simulink model "PID_Tune"  (R2021b)
settings: Solver=FixedStepAuto  StartTime=0.0  StopTime=20  FixedStep=0.1  RelTol=1e-3
values from neighbouring files (symbols this model uses):
  inner_h = 0.1    [dataset.mat]    (also in initiateVars.m; system_workspace.mat; system_workspace_ayk.mat)
  omega_max_lim = 2500    [dataset.mat]    (also in initiateVars.m; system_workspace.mat; system_workspace_ayk.mat)
  omega_min_lim = 0    [dataset.mat]    (also in initiateVars.m; system_workspace.mat; system_workspace_ayk.mat)
  T_max_lim = 0.495    [dataset.mat]    (also in initiateVars.m = Tp - (Tp - Tm) * sat_lim; system_workspace.mat; system_workspace_ayk.mat)
  T_min_lim = 0.055    [dataset.mat]    (also in initiateVars.m = Tm + (Tp - Tm) * sat_lim; system_workspace.mat; system_workspace_ayk.mat)
  tau_max_lim = 1e-05    [dataset.mat]    (also in initiateVars.m; system_workspace.mat; system_workspace_ayk.mat)
  tau_min_lim = -1e-05    [dataset.mat]    (also in initiateVars.m; system_workspace.mat; system_workspace_ayk.mat)
libraries: slpidlib x2
settings Model: Creator=fethi  LastModifiedBy=fethi
settings SolverCC: AlgebraicLoopSolver=TrustRegion
settings DebuggingCC: SFMachineParentedDataDiag=warning

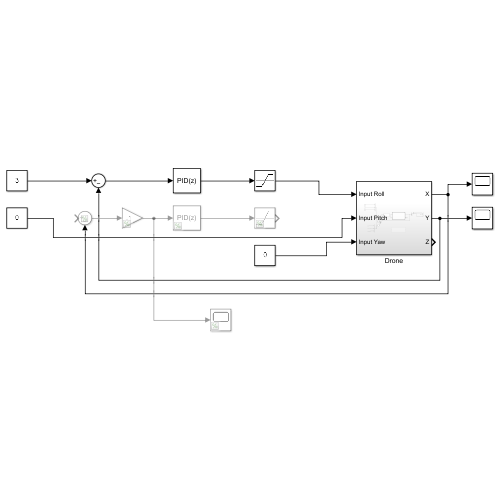
[thumbnail: Simulink's stored preview of the top-level diagram]
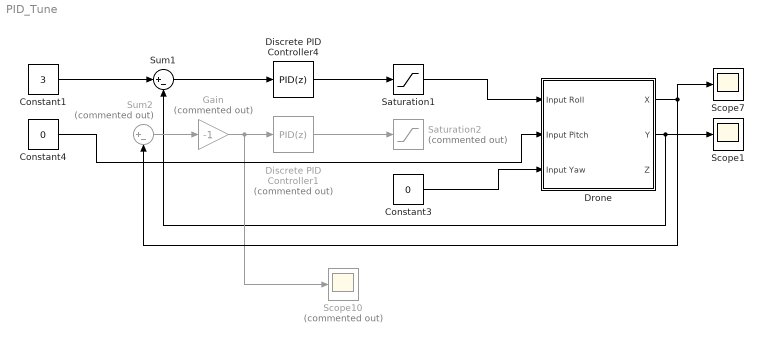
== system PID_Tune ==
  Constant1 : Constant  Value=3
  Constant3 : Constant  Value=0
  Constant4 : Constant  Value=0
  Discrete PID Controller1 : slpidlib/PID Controller  Commented=on  Controller=PID  Form=Parallel  TimeDomain=Discrete-time  UseExternalTs=off  SampleTime=-1  IntegratorMethod=Forward Euler  FilterMethod=Forward Euler  ControllerParametersSource=internal  P=-0.034  I=-8.37942170328314e-06  D=-0.0838262219971284  UseFilter=on  N=16.4387565401463  TunerSelectOption=Transfer Function Based (PID Tuner App)  InitialConditionSource=internal  InitialConditionForIntegrator=0  InitialConditionForFilter=0  DifferentiatorICPrevScaledInput=0  ExternalReset=none  TrackingMode=off  Kt=1  LimitOutput=off  SatLimitsSource=internal  UpperSaturationLimit=inf  LowerSaturationLimit=-inf  LinearizeAsGain=off  AntiWindupMode=none  Kb=1  POutMin=[]  POutMax=[]  IOutMin=[]  IOutMax=[]  DOutMin=[]  DOutMax=[]  NOutMin=[]  NOutMax=[]  SumOutMin=[]  SumOutMax=[]  SaturationOutMin=[]  SaturationOutMax=[]  PParamMin=[]  PParamMax=[]  IParamMin=[]  IParamMax=[]  DParamMin=[]  DParamMax=[]  NParamMin=[]  NParamMax=[]  KbParamMin=[]  KbParamMax=[]  KtParamMin=[]  KtParamMax=[]  KbOutMin=[]  KbOutMax=[]  KtOutMin=[]  KtOutMax=[]  IntegratorOutMin=[]  IntegratorOutMax=[]  FilterOutMin=[]  FilterOutMax=[]  SumI1OutMin=[]  SumI1OutMax=[]  SumI2OutMin=[]  SumI2OutMax=[]  SumI3OutMin=[]  SumI3OutMax=[]  SumI4OutMin=[]  SumI4OutMax=[]  SumDOutMin=[]  SumDOutMax=[]  DifferentiatorOutMin=[]  DifferentiatorOutMax=[]  FilterDiffOutCoefMin=[]  FilterDiffOutCoefMax=[]  ReciprocalOutMin=[]  ReciprocalOutMax=[]  SumDenOutMin=[]  SumDenOutMax=[]  SumNumOutMin=[]  SumNumOutMax=[]  DivideOutMin=[]  DivideOutMax=[]  UdiffTsProdOutMin=[]  UdiffTsProdOutMax=[]  NTsProdOutMin=[]  NTsProdOutMax=[]  UintegralTsProdOutMin=[]  UintegralTsProdOutMax=[]  UngainTsProdOutMin=[]  UngainTsProdOutMax=[]  IntegratorContinuousStateAttributes=''  IntegratorStateMustResolveToSignalObject=off  IntegratorRTWStateStorageClass=Auto  FilterContinuousStateAttributes=''  FilterStateMustResolveToSignalObject=off  FilterRTWStateStorageClass=Auto  ParallelPVariant=InternalParameters  IdealPVariant=Disabled  IVariant=InternalParameters  DVariant=InternalParameters  IntegratorVariant=Discrete  SatVariant=Disabled  AWVariant=Passthrough  PCopyVariant=Disabled  TRVariant=Disabled  FdbkBlocksVariant=Forward  IdealPFdbkVariant=Disabled  SatFdbkVariant=Disabled  DerivativeFilterVariant=ForwardEulerFilter  NVariant=InternalParameters  NCopyVariant=Disabled  FilterICVariant=InternalICsFilter  IntegratorICVariant=InternalICs  ExternalResetVariant=Disabled  TRSumVariant=Passthrough  SumFdbkVariant=Disabled  SumVariant=Sum_PID  TsampFilterVariant=InternalTs  TsampNgainVariant=Passthrough  TsampIntegralVariant=Passthrough  ExternalSaturationOutDataTypeStr=Inherit: Same as second input
  Discrete PID Controller4 : slpidlib/PID Controller  Controller=PID  Form=Parallel  TimeDomain=Discrete-time  UseExternalTs=off  SampleTime=-1  IntegratorMethod=Forward Euler  FilterMethod=Forward Euler  ControllerParametersSource=internal  P=-0.034  I=-8.37942170328314e-06  D=-0.0838262219971284  UseFilter=on  N=16.4387565401463  TunerSelectOption=Transfer Function Based (PID Tuner App)  InitialConditionSource=internal  InitialConditionForIntegrator=0  InitialConditionForFilter=0  DifferentiatorICPrevScaledInput=0  ExternalReset=none  TrackingMode=off  Kt=1  LimitOutput=off  SatLimitsSource=internal  UpperSaturationLimit=inf  LowerSaturationLimit=-inf  LinearizeAsGain=off  AntiWindupMode=none  Kb=1  POutMin=[]  POutMax=[]  IOutMin=[]  IOutMax=[]  DOutMin=[]  DOutMax=[]  NOutMin=[]  NOutMax=[]  SumOutMin=[]  SumOutMax=[]  SaturationOutMin=[]  SaturationOutMax=[]  PParamMin=[]  PParamMax=[]  IParamMin=[]  IParamMax=[]  DParamMin=[]  DParamMax=[]  NParamMin=[]  NParamMax=[]  KbParamMin=[]  KbParamMax=[]  KtParamMin=[]  KtParamMax=[]  KbOutMin=[]  KbOutMax=[]  KtOutMin=[]  KtOutMax=[]  IntegratorOutMin=[]  IntegratorOutMax=[]  FilterOutMin=[]  FilterOutMax=[]  SumI1OutMin=[]  SumI1OutMax=[]  SumI2OutMin=[]  SumI2OutMax=[]  SumI3OutMin=[]  SumI3OutMax=[]  SumI4OutMin=[]  SumI4OutMax=[]  SumDOutMin=[]  SumDOutMax=[]  DifferentiatorOutMin=[]  DifferentiatorOutMax=[]  FilterDiffOutCoefMin=[]  FilterDiffOutCoefMax=[]  ReciprocalOutMin=[]  ReciprocalOutMax=[]  SumDenOutMin=[]  SumDenOutMax=[]  SumNumOutMin=[]  SumNumOutMax=[]  DivideOutMin=[]  DivideOutMax=[]  UdiffTsProdOutMin=[]  UdiffTsProdOutMax=[]  NTsProdOutMin=[]  NTsProdOutMax=[]  UintegralTsProdOutMin=[]  UintegralTsProdOutMax=[]  UngainTsProdOutMin=[]  UngainTsProdOutMax=[]  IntegratorContinuousStateAttributes=''  IntegratorStateMustResolveToSignalObject=off  IntegratorRTWStateStorageClass=Auto  FilterContinuousStateAttributes=''  FilterStateMustResolveToSignalObject=off  FilterRTWStateStorageClass=Auto  ParallelPVariant=InternalParameters  IdealPVariant=Disabled  IVariant=InternalParameters  DVariant=InternalParameters  IntegratorVariant=Discrete  SatVariant=Disabled  AWVariant=Passthrough  PCopyVariant=Disabled  TRVariant=Disabled  FdbkBlocksVariant=Forward  IdealPFdbkVariant=Disabled  SatFdbkVariant=Disabled  DerivativeFilterVariant=ForwardEulerFilter  NVariant=InternalParameters  NCopyVariant=Disabled  FilterICVariant=InternalICsFilter  IntegratorICVariant=InternalICs  ExternalResetVariant=Disabled  TRSumVariant=Passthrough  SumFdbkVariant=Disabled  SumVariant=Sum_PID  TsampFilterVariant=InternalTs  TsampNgainVariant=Passthrough  TsampIntegralVariant=Passthrough  ExternalSaturationOutDataTypeStr=Inherit: Same as second input
  Drone : Subsystem
  Gain : Gain  Commented=on  Gain=-1
  Saturation1 : Saturate  UpperLimit=pi/18  LowerLimit=-pi/18
  Saturation2 : Saturate  Commented=on  UpperLimit=pi/18  LowerLimit=-pi/18
  Scope1 : Scope
  Scope10 : Scope  Commented=on
  Scope7 : Scope
  Sum1 : Sum  Inputs=|+-
  Sum2 : Sum  Commented=on  Inputs=|+-
  wires:
  Constant3/1 -> Drone/3(Input Yaw)
  Constant1/1 -> Sum1/1
  Sum1/1 -> Discrete PID Controller4/1
  Discrete PID Controller4/1 -> Saturation1/1
  Discrete PID Controller1/1 -> Saturation2/1
  Drone/2(Y) -> Scope1/1, Sum1/2
  Sum2/1 -> Gain/1
  Gain/1 -> Discrete PID Controller1/1, Scope10/1
  Drone/1(X) -> Sum2/2, Scope7/1
  Saturation1/1 -> Drone/1(Input Roll)
  Constant4/1 -> Drone/2(Input Pitch)

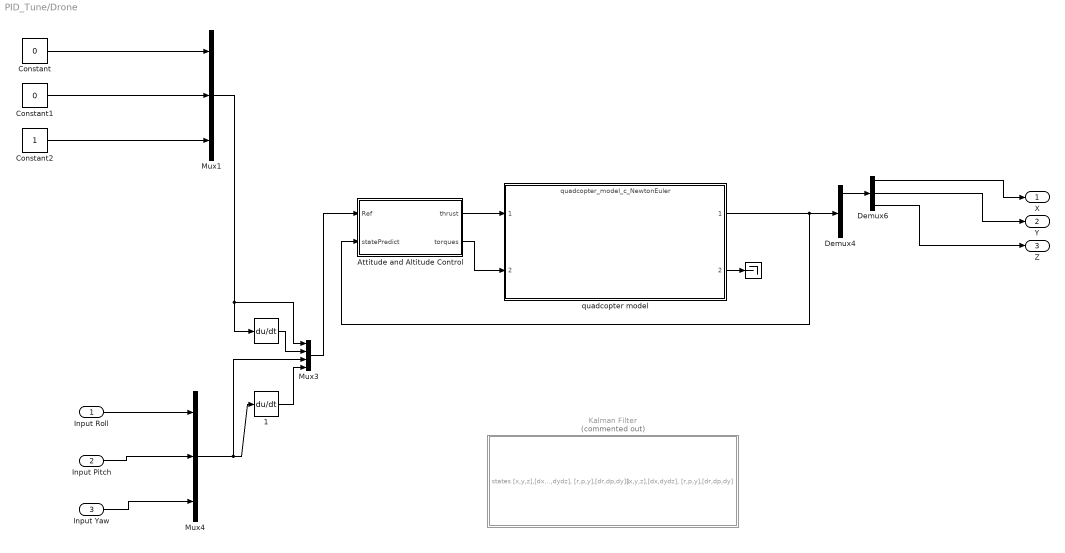
== system PID_Tune/Drone ==
  Input Roll : Inport
  Input Pitch : Inport  Port=2
  Input Yaw : Inport  Port=3
  "   " : Terminator
  "        " : Derivative
  "        1" : Derivative
  Attitude and Altitude Control : Subsystem
  Constant : Constant  Value=0
  Constant1 : Constant  Value=0
  Constant2 : Constant
  Demux4 : Demux  Outputs=[3,3,3,3]
  Demux6 : Demux  Outputs=[1,1,1]
  Kalman Filter : Subsystem  Commented=on
  Mux1 : Mux  Inputs=3
  Mux3 : Mux
  Mux4 : Mux  Inputs=3
  quadcopter model : ModelReference  ModelNameDialog=quadcopter_model_c_NewtonEuler.mdl  SimulationMode=Normal  ModelReferenceVersion=1.355
  X : Outport
  Y : Outport  Port=2
  Z : Outport  Port=3
  wires:
  Demux6/3 -> Z/1
  Demux6/2 -> Y/1
  Demux6/1 -> X/1
  Attitude and Altitude Control/2(torques) -> quadcopter model/2
  quadcopter model/2 -> "   "/1
  Attitude and Altitude Control/1(thrust) -> quadcopter model/1
  quadcopter model/1 -> Demux4/1, Attitude and Altitude Control/2(statePredict)
  Demux4/1 -> Demux6/1
  Mux1/1 -> Mux3/1, "        "/1
  Input Pitch/1 -> Mux4/2
  Constant2/1 -> Mux1/3
  Input Yaw/1 -> Mux4/3
  Input Roll/1 -> Mux4/1
  "        "/1 -> Mux3/2
  Constant1/1 -> Mux1/2
  Constant/1 -> Mux1/1
  Mux3/1 -> Attitude and Altitude Control/1(Ref)
  "        1"/1 -> Mux3/4
  Mux4/1 -> "        1"/1, Mux3/3

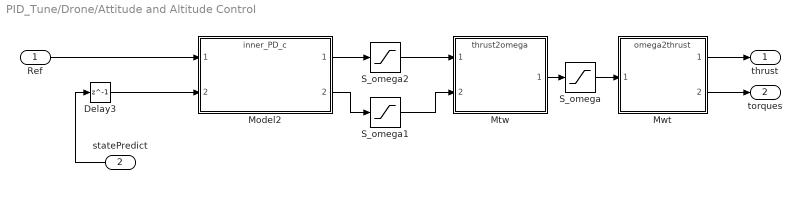
== system PID_Tune/Drone/Attitude and Altitude Control ==
  Ref : Inport
  statePredict : Inport  Port=2
  Delay3 : Delay  DelayLength=1  InitialCondition=0  SampleTime=inner_h
  Model2 : ModelReference  ModelNameDialog=inner_PD_c.mdl  SimulationMode=Normal  ModelReferenceVersion=1.90
  Mtw : ModelReference  ModelNameDialog=thrust2omega.mdl  SimulationMode=Normal  ModelReferenceVersion=1.7
  Mwt : ModelReference  ModelNameDialog=omega2thrust.mdl  SimulationMode=Normal  ModelReferenceVersion=1.7
  S_omega : Saturate  UpperLimit=omega_max_lim  LowerLimit=omega_min_lim
  S_omega1 : Saturate  UpperLimit=tau_max_lim  LowerLimit=tau_min_lim
  S_omega2 : Saturate  UpperLimit=T_max_lim  LowerLimit=T_min_lim
  thrust : Outport  VectorParamsAs1DForOutWhenUnconnected=off
  torques : Outport  Port=2  VectorParamsAs1DForOutWhenUnconnected=off
  wires:
  statePredict/1 -> Delay3/1
  Mwt/2 -> torques/1
  Ref/1 -> Model2/1
  Delay3/1 -> Model2/2
  Model2/2 -> S_omega1/1
  Mwt/1 -> thrust/1
  Model2/1 -> S_omega2/1
  Mtw/1 -> S_omega/1
  S_omega2/1 -> Mtw/1
  S_omega1/1 -> Mtw/2
  S_omega/1 -> Mwt/1

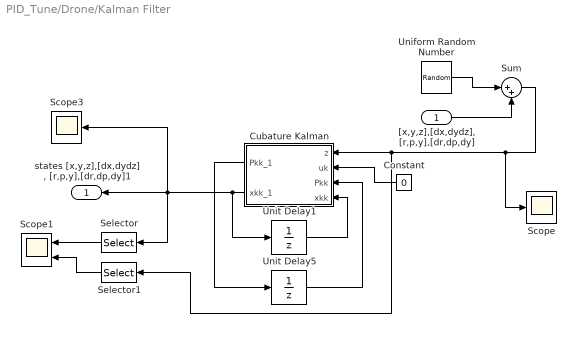
== system PID_Tune/Drone/Kalman Filter ==
  "[x,y,z],[dx,dydz], [r,p,y],[dr,dp,dy]" : Inport
  Constant : Constant  Value=0
  Cubature Kalman : MATLAB Function  TreatAsAtomicUnit=on
  Scope : Scope
  Scope1 : Scope  NumInputPorts=2
  Scope3 : Scope
  Selector : Selector  InputPortWidth=12  IndexOptions=Index vector (dialog)  Indices=[3]  OutputSizes=1
  Selector1 : Selector  InputPortWidth=12  IndexOptions=Index vector (dialog)  Indices=[3]  OutputSizes=1
  Sum : Sum  Inputs=|++
  Uniform Random Number : UniformRandomNumber  Minimum=-0.001  Maximum=0.001  SampleTime=0.1
  Unit Delay1 : UnitDelay  InitialCondition=[0 0 0 0 0 0 0 0 0 0 0 0]  SampleTime=-1  HasFrameUpgradeWarning=on
  Unit Delay5 : UnitDelay  InitialCondition=eye(12)*10^-3  SampleTime=-1  HasFrameUpgradeWarning=on
  "states [x,y,z],[dx,dydz], [r,p,y],[dr,dp,dy]1" : Outport  PortDimensions=12  VectorParamsAs1DForOutWhenUnconnected=off
  wires:
  "[x,y,z],[dx,dydz], [r,p,y],[dr,dp,dy]"/1 -> Sum/2
  Uniform Random Number/1 -> Sum/1
  Sum/1 -> Scope/1, Cubature Kalman/1(z), Selector1/1
  Selector1/1 -> Scope1/2
  Selector/1 -> Scope1/1
  Unit Delay1/1 -> Cubature Kalman/4(xkk)
  Cubature Kalman/2(xkk_1) -> Unit Delay1/1, Scope3/1, "states [x,y,z],[dx,dydz], [r,p,y],[dr,dp,dy]1"/1, Selector/1
  Constant/1 -> Cubature Kalman/2(uk)
  Cubature Kalman/1(Pkk_1) -> Unit Delay5/1
  Unit Delay5/1 -> Cubature Kalman/3(Pkk)

== matlab function PID_Tune/Drone/Kalman Filter/Cubature Kalman ==
  data: Pkk_1 output; z input; uk input; Pkk input; xkk input; xkk_1 output
function [Pkk_1, xkk_1]   = fcn(z, uk, Pkk, xkk)

%% Model
A = 1;
B = 0;

%% Covariances
Q = diag([0.1 0.1 0.1 0.1 0.1 0.1 0.1 0.1 0.1 0.1 0.1 0.1])*100;
R = 0.01;   
% gyro = z(4:6);
% delta = [1*(gyro'-xkk(4:6));0;0;0;0];
% z1 = [z(1:3)' - xkk(1:3); z(1:3)' - xkk(1:3); z(7)];  
%% Cubature Kalman Predict
xkk1 = A*xkk ;
Pkk1 = A*Pkk*A' + Q; 

%% Cubature Kalman Update
%%%========================================================================
%%% Genrate a set of Cubature Points
%%%========================================================================

nx = 12; % state vector dimension

nPts = 2*nx;   % No. of Cubature Points

CPtArray = sqrt(nPts/2)*[eye(nx) -eye(nx)];

%%%========================================================================
%%% find the square-root of Pkk1 using Singular Value Decomposition (SVD)
%%%========================================================================

Pkk1 = 0.5*(Pkk1+Pkk1'); % make Pkk1 to be symmetric (Property of a covariance matrix !)

[U, S, V] =  svd(Pkk1);

Skk1 = 0.5*(U+V)*sqrt(S);

%%%========================================================================

Xi =  repmat(xkk1,1,nPts) + Skk1*CPtArray;

% Zi = Zi1(1,:);
% Zi = cartpend(Xi,uk, Zi1);
% bias = [0.00017;0.00017;0.00017;0.00076;0.00076;0.00076;0.001]; 
% bias = repmat(bias,1,14);
Zi = Xi;
% Zi = Zi1';

    

zkk1 = sum(Zi,2)/nPts;      % predicted Measurement

X = (Xi-repmat(xkk1,1,nPts))/sqrt(nPts);
    
Z = (Zi-repmat(zkk1,1,nPts))/sqrt(nPts);  

Pzz = Z*Z'+ R; % Innovations Covariance

Pxz = X*Z'; % cross-covariance
    
G = Pxz*pinv(Pzz);         % Cubature Kalman Gain  
    
xkk_1 = xkk1 + G*(z - zkk1);  

Pkk_1 = Pkk1 - G*Pzz*G';
